simulink model "model2_inout"  (R2021b)
settings: Solver=VariableStepAuto  StartTime=0.0  StopTime=10.0  RelTol=1e-3
settings Model: Creator=AMY  LastModifiedBy=AMY

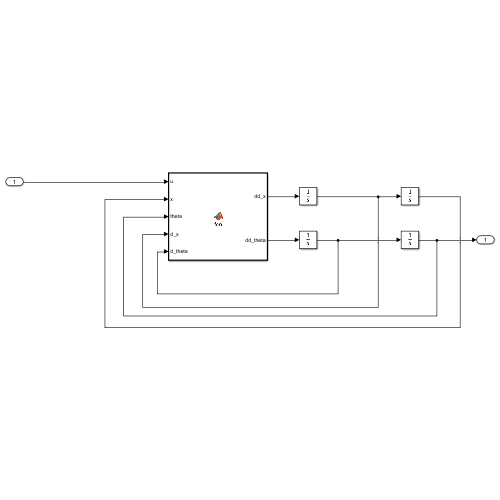
[thumbnail: Simulink's stored preview of the top-level diagram]
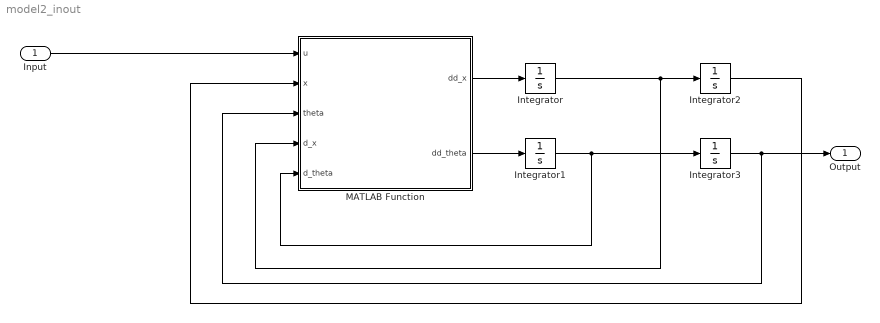
== system model2_inout ==
  Input : Inport
  Integrator{,1..3} (4 alike) : Integrator
  MATLAB Function : MATLAB Function  TreatAsAtomicUnit=on
  Output : Outport
  wires:
  MATLAB Function/2(dd_theta) -> Integrator1/1
  Integrator/1 -> MATLAB Function/4(d_x), Integrator2/1
  Integrator3/1 -> Output/1, MATLAB Function/3(theta)
  Input/1 -> MATLAB Function/1(u)
  Integrator1/1 -> Integrator3/1, MATLAB Function/5(d_theta)
  Integrator2/1 -> MATLAB Function/2(x)
  MATLAB Function/1(dd_x) -> Integrator/1

== matlab function model2_inout/MATLAB Function ==
  data: dd_x output; u input; dd_theta output; x input; theta input; d_x input; d_theta input
function [dd_x, dd_theta] = fcn(u, x, theta,  d_x, d_theta)

    m = 1.5;          %Masa corpului
    g = 9.81;         %Acceleratia gravitationala
    zeta = 0.6;      %Coeficient de amortizare
    k = 1.5;          %Constanta elastica
    l0 = 0.5;         %Lungimea initiala a resortului
    
    %Ecuatiile
    dd_x = (l0+x)*(d_theta)*(d_theta) - (k/m)*x + g*cos(theta) - zeta*d_x;
    dd_theta = -(g/(l0+x)*sin(theta))-(2*d_x/(l0+x))*d_theta - zeta*d_theta + 1/(m*(l0+x)*(l0+x))*u;

end
